simulink model "fa"  (R2020a)
settings: Solver=VariableStepAuto  StartTime=0.0  StopTime=10.0  RelTol=1e-3
settings Model: Creator=kishan  LastModifiedBy=kishan

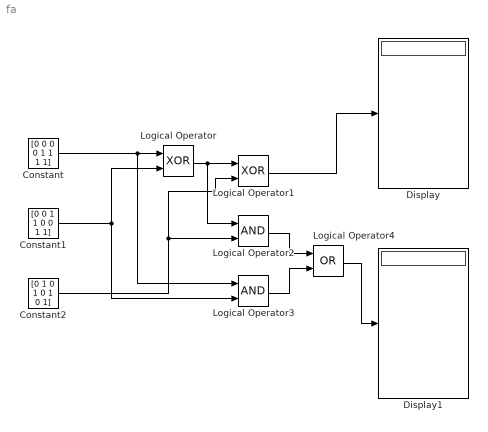
== system fa ==
  Constant : Constant  Value=[0 0 0 0 1 1 1 1]
  Constant1 : Constant  Value=[0 0 1 1 0 0 1 1]
  Constant2 : Constant  Value=[0 1 0 1 0 1 0 1]
  Display : Display
  Display1 : Display
  Logical Operator : Logic  Operator=XOR  AllPortsSameDT=off  OutDataTypeStr=boolean
  Logical Operator1 : Logic  Operator=XOR  AllPortsSameDT=off  OutDataTypeStr=boolean
  Logical Operator2 : Logic  AllPortsSameDT=off  OutDataTypeStr=boolean
  Logical Operator3 : Logic  AllPortsSameDT=off  OutDataTypeStr=boolean
  Logical Operator4 : Logic  Operator=OR  AllPortsSameDT=off  OutDataTypeStr=boolean
  wires:
  Logical Operator2/1 -> Logical Operator4/1
  Logical Operator3/1 -> Logical Operator4/2
  Logical Operator/1 -> Logical Operator2/1, Logical Operator1/1
  Constant/1 -> Logical Operator3/1, Logical Operator/1
  Constant1/1 -> Logical Operator3/2, Logical Operator/2
  Constant2/1 -> Logical Operator2/2, Logical Operator1/2
  Logical Operator1/1 -> Display/1
  Logical Operator4/1 -> Display1/1
